simulink model "BackwardAccConverter"  (R2023a)
settings: Solver=VariableStepAuto  StartTime=0.0  StopTime=10.0  RelTol=1e-3
settings Model: Creator=Waffle  LastModifiedBy=Waffle

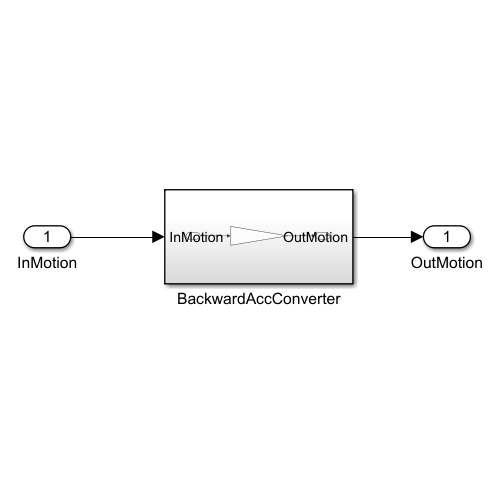
[thumbnail: Simulink's stored preview of the top-level diagram]
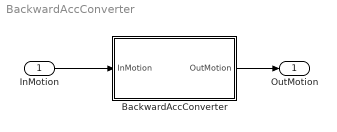
== system BackwardAccConverter ==
  InMotion : Inport
  BackwardAccConverter : Subsystem
  OutMotion : Outport
  wires:
  InMotion/1 -> BackwardAccConverter/1(InMotion)
  BackwardAccConverter/1(OutMotion) -> OutMotion/1

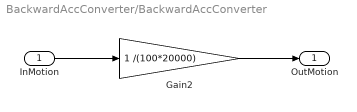
== system BackwardAccConverter/BackwardAccConverter ==
  InMotion : Inport
  Gain2 : Gain  Gain=1 /(100*20000)
  OutMotion : Outport
  wires:
  InMotion/1 -> Gain2/1
  Gain2/1 -> OutMotion/1
